simulink model "CancerImmunology"  (Simulink 8.6)
settings: Solver=ode8  StartTime=0.0  StopTime=1  FixedStep=0.001  RelTol=1e-3
settings Model: Creator=MAHDI  LastModifiedBy=MAHDI
settings DataIOCC: SaveFormat=Dataset  SignalLoggingSaveFormat=Dataset
settings OptimizationCC: ExpressionDepthLimit=128
settings DebuggingCC: UnderspecifiedInitializationDetection=Simplified  MergeDetectMultiDrivingBlocksExec=error  SolverPrmCheckMsg=none  FcnCallInpInsideContextMsg=EnableAllAsError  StateNameClashWarn=none
settings HardwareCC: ProdBitPerPointer=64  ProdLargestAtomicFloat=Float  ProdIntDivRoundTo=Zero  ProdEndianess=LittleEndian  ProdWordSize=64  ProdHWDeviceType=Intel->x86-64 (Windows64)
settings GRTTargetCC: GeneratePreprocessorConditionals=Use local settings  CombineOutputUpdateFcns=on  GRTInterface=off
settings ConfigComp: CovModelRefEnable=off

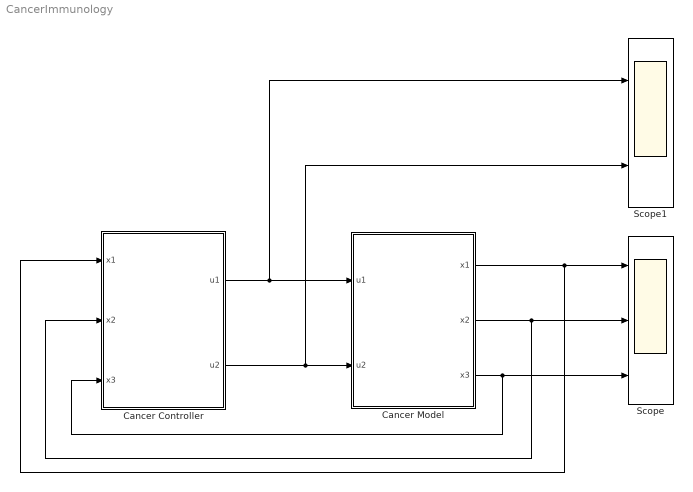
== system CancerImmunology ==
  Cancer Controller : Subsystem
  Cancer Model : Subsystem
  Scope : Scope  NumInputPorts=3
  Scope1 : Scope  NumInputPorts=2
  wires:
  Cancer Controller/1(u1) -> Scope1/1, Cancer Model/1(u1)
  Cancer Controller/2(u2) -> Cancer Model/2(u2), Scope1/2
  Cancer Model/1(x1) -> Cancer Controller/1(x1), Scope/1
  Cancer Model/2(x2) -> Cancer Controller/2(x2), Scope/2
  Cancer Model/3(x3) -> Cancer Controller/3(x3), Scope/3

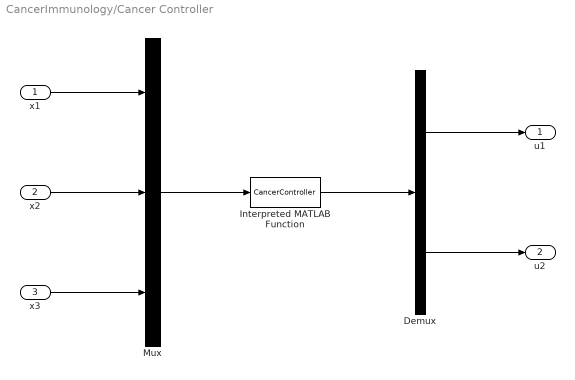
== system CancerImmunology/Cancer Controller ==
  x1 : Inport
  x2 : Inport  Port=2
  x3 : Inport  Port=3
  Demux : Demux  Outputs=2
  Interpreted MATLAB Function : MATLABFcn  MATLABFcn=CancerController  OutputDimensions=2
  Mux : Mux  Inputs=3
  u1 : Outport
  u2 : Outport  Port=2
  wires:
  Interpreted MATLAB Function/1 -> Demux/1
  Mux/1 -> Interpreted MATLAB Function/1
  x1/1 -> Mux/1
  x2/1 -> Mux/2
  x3/1 -> Mux/3
  Demux/1 -> u1/1
  Demux/2 -> u2/1

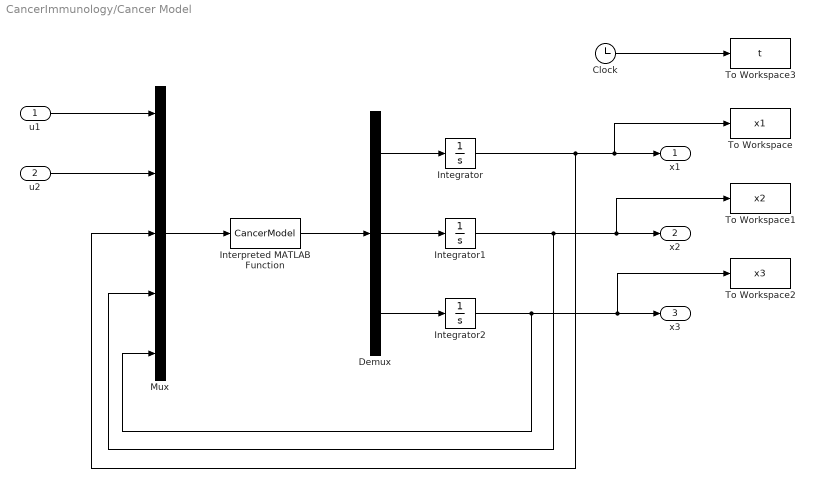
== system CancerImmunology/Cancer Model ==
  u1 : Inport
  u2 : Inport  Port=2
  Clock : Clock
  Demux : Demux  Outputs=3
  Integrator : Integrator  InitialCondition=180000
  Integrator1 : Integrator  InitialCondition=1.2
  Integrator2 : Integrator  InitialCondition=9.8
  Interpreted MATLAB Function : MATLABFcn  MATLABFcn=CancerModel  OutputDimensions=3
  Mux : Mux  Inputs=5
  To Workspace : ToWorkspace  VariableName=x1  SampleTime=-1
  To Workspace1 : ToWorkspace  VariableName=x2  SampleTime=-1
  To Workspace2 : ToWorkspace  VariableName=x3  SampleTime=-1
  To Workspace3 : ToWorkspace  VariableName=t  SampleTime=-1
  x1 : Outport
  x2 : Outport  Port=2
  x3 : Outport  Port=3
  wires:
  Demux/2 -> Integrator1/1
  Demux/1 -> Integrator/1
  Demux/3 -> Integrator2/1
  Integrator/1 -> Mux/3, To Workspace/1, x1/1
  Integrator1/1 -> Mux/4, To Workspace1/1, x2/1
  Integrator2/1 -> Mux/5, To Workspace2/1, x3/1
  Interpreted MATLAB Function/1 -> Demux/1
  Mux/1 -> Interpreted MATLAB Function/1
  u1/1 -> Mux/1
  u2/1 -> Mux/2
  Clock/1 -> To Workspace3/1
